simulink model "inverted_pendulum"  (R2020a)
settings: Solver=VariableStepAuto  StartTime=0.0  StopTime=10.0  RelTol=1e-3
settings Model: Creator=sidsu  LastModifiedBy=sidsu

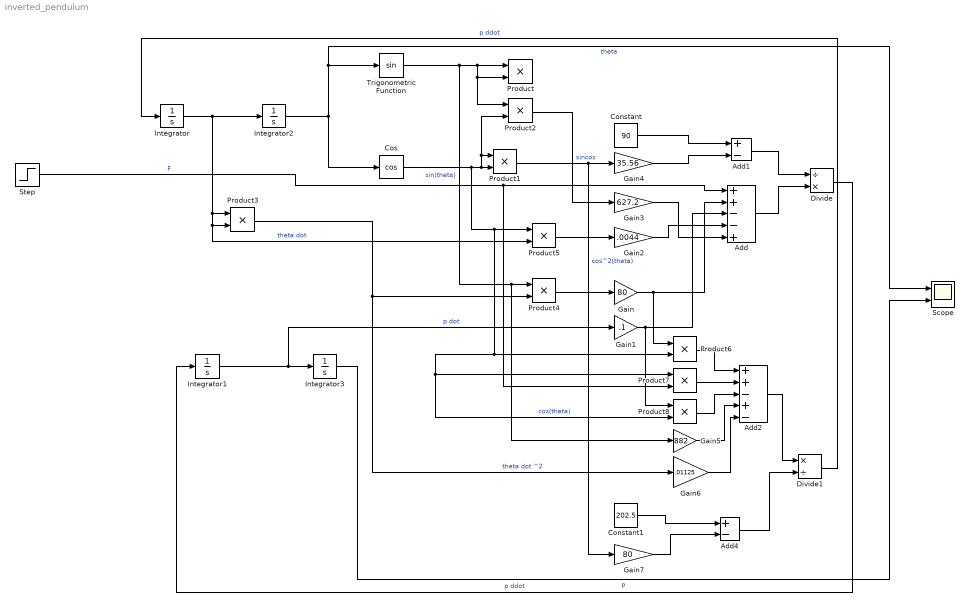
== system inverted_pendulum ==
  Add : Sum  Inputs=++--+
  Add1 : Sum  Inputs=+-
  Add2 : Sum  Inputs=++-+-
  Add4 : Sum  Inputs=+-
  Constant : Constant  Value=90
  Constant1 : Constant  Value=202.5
  Cos : Trigonometry  Operator=cos
  Divide : Product  Inputs=/*
  Divide1 : Product  Inputs=*/
  Gain : Gain  Gain=80
  Gain1 : Gain  Gain=.1
  Gain2 : Gain  Gain=.0044
  Gain3 : Gain  Gain=627.2
  Gain4 : Gain  Gain=35.56
  Gain5 : Gain  Gain=882
  Gain6 : Gain  Gain=.01125
  Gain7 : Gain  Gain=80
  Integrator{,1..3} (4 alike) : Integrator
  Product{,1..8} (9 alike) : Product
  Scope : Scope  NumInputPorts=2
  Step : Step  SampleTime=0
  Trigonometric Function : Trigonometry
  wires:
  Integrator1/1 -> Gain1/1, Integrator3/1  "p dot"
  Integrator/1 -> Product5/2, Product3/2, Product3/1, Integrator2/1  "theta dot"
  Integrator2/1 -> Cos/1, Scope/1, Trigonometric Function/1  "theta"
  Integrator3/1 -> Scope/2  "p"
  Divide/1 -> Integrator1/1  "p ddot"
  Trigonometric Function/1 -> Gain5/1, Product4/1, Product2/1, Product/2, Product/1  "sin(theta)"
  Cos/1 -> Product8/2, Product7/1, Product6/2, Product5/1, Product2/2, Product1/1, Product1/2  "cos(theta)"
  Product1/1 -> Gain7/1, Gain4/1  "cos^2(theta)"
  Product2/1 -> Gain3/1  "sincos"
  Product3/1 -> Gain6/1, Product4/2  "theta dot ^2"
  Step/1 -> Add/1, Product7/2  "F"
  Product4/1 -> Gain/1
  Product5/1 -> Gain2/1
  Gain/1 -> Add/2, Product6/1
  Gain2/1 -> Add/4
  Gain3/1 -> Add/5
  Constant/1 -> Add1/1
  Gain4/1 -> Add1/2
  Add/1 -> Divide/2
  Add1/1 -> Divide/1
  Gain1/1 -> Add/3, Product8/1
  Product7/1 -> Add2/2
  Product6/1 -> Add2/1
  Product8/1 -> Add2/3
  Gain5/1 -> Add2/4
  Gain6/1 -> Add2/5
  Gain7/1 -> Add4/2
  Constant1/1 -> Add4/1
  Add2/1 -> Divide1/1
  Add4/1 -> Divide1/2
  Divide1/1 -> Integrator/1  "p ddot"
